simulink model "washing_machine_chart"  (R2024b)
settings: Solver=VariableStepAuto  StartTime=0.0  StopTime=inf  RelTol=1e-3
settings Model: Creator=heman  LastModifiedBy=heman

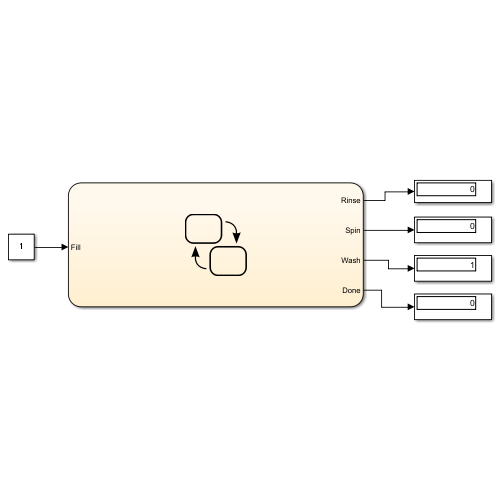
[thumbnail: Simulink's stored preview of the top-level diagram]
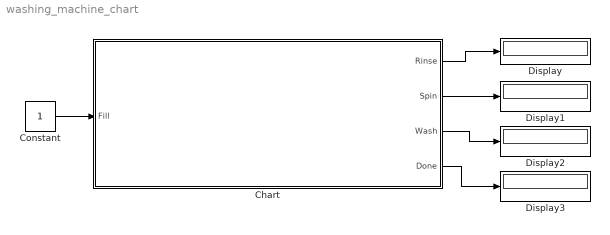
== system washing_machine_chart ==
  Chart : Stateflow chart  TreatAsAtomicUnit=on
  Constant : Constant
  Display{,1..3} (4 alike) : Display
  wires:
  Constant/1 -> Chart/1(Fill)
  Chart/2(Spin) -> Display1/1
  Chart/1(Rinse) -> Display/1
  Chart/4(Done) -> Display3/1
  Chart/3(Wash) -> Display2/1

== stateflow chart washing_machine_chart/Chart ==
  state Fill
    entry:Fill==1;
  state Wash
    entry:Wash=1;
  state Rinse
    entry:Rinse=1;
  state Spin
    entry:Spin=1;
  state Done
    entry:Done=1;
  (default) -> Fill
  Fill -> Wash : [after(10,sec)]
  Wash -> Rinse : after(40,sec)
  Rinse -> Spin : after(40,sec)
  Spin -> Done : after(40,sec)
  data: Rinse output double; Spin output double; Wash output double; Done output; Fill input
